simulink model "ford_expedition_cosimulation"  (R2021b)
settings: Solver=ode45  StartTime=0.0  StopTime=45  FixedStep=0.01  RelTol=1e-3  EnableMultiTasking=on
libraries: instrumentlib x2, slpidlib x1
settings Model: PacingRate=11  Creator=tasora  LastModifiedBy=Trevor
settings SolverCC: AlgebraicLoopSolver=TrustRegion
settings DataIOCC: LimitDataPoints=on  SaveFormat=Array  SignalLoggingSaveFormat=ModelDataLogs  ReturnWorkspaceOutputs=off
settings OptimizationCC: ExpressionDepthLimit=2147483647  LifeSpan=inf
settings DebuggingCC: UnderspecifiedInitializationDetection=Classic  MergeDetectMultiDrivingBlocksExec=none  SolverPrmCheckMsg=warning  FcnCallInpInsideContextMsg=warning  StateNameClashWarn=warning  SFUnexpectedBacktrackingDiag=warning  SFNoUnconditionalDefaultTransitionDiag=warning  SFExecutionAtInitializationDiag=none  SFMachineParentedDataDiag=warning  ArithmeticOperatorsInVariantConditions=warning
settings HardwareCC: ProdBitPerPointer=32  ProdBitPerSizeT=32  ProdBitPerPtrDiffT=32  ProdLargestAtomicFloat=None  ProdIntDivRoundTo=Undefined  ProdEndianess=Unspecified  ProdWordSize=32  ProdHWDeviceType=32-bit Generic
settings ModelReferenceCC: PropagateSignalLabelsOutOfModel=off
settings SFSimCC: SimUseLocalCustomCode=off  CustomCodeUndefinedFunction=UseInterfaceOnly
settings RTWCC: RTWUseLocalCustomCode=off
settings CodeAppCC: StateflowObjectComments=on
settings GRTTargetCC: TargetLangStandard=C89/C90 (ANSI)  CombineOutputUpdateFcns=off  GRTInterface=on
settings ConfigComp: CovMetricSettings=dw  CovSaveCumulativeToWorkspaceVar=on  CovSaveSingleToWorkspaceVar=on  CovExternalEMLEnable=off

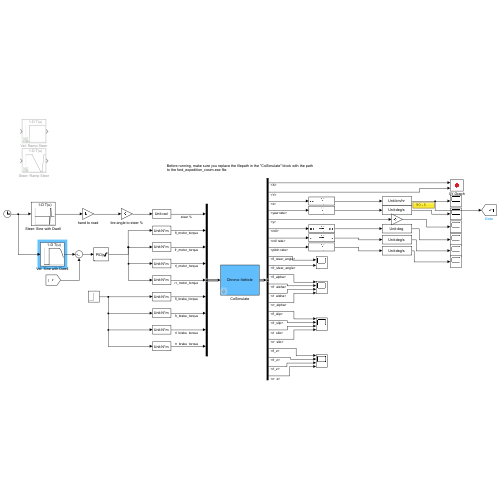
[thumbnail: Simulink's stored preview of the top-level diagram]
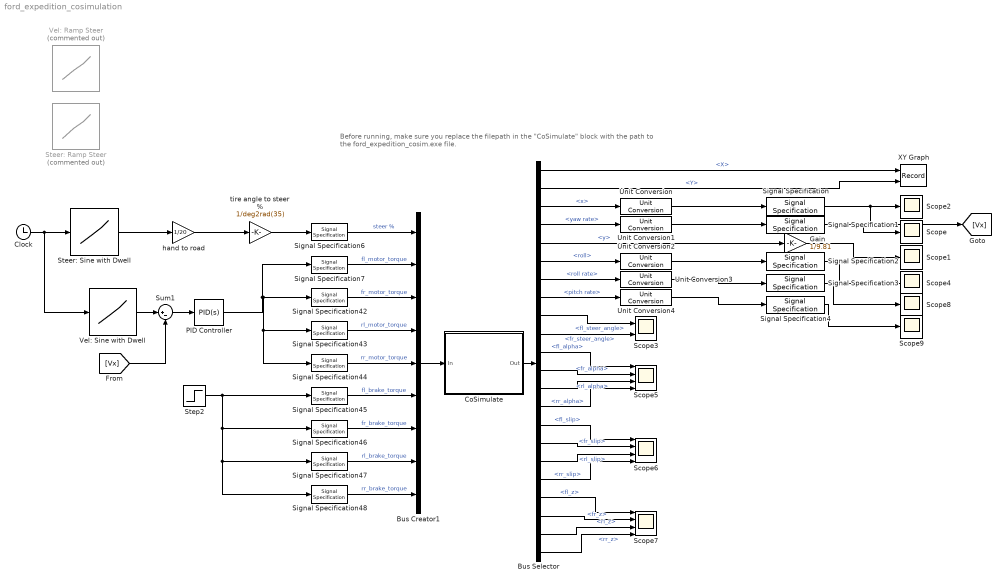
== system ford_expedition_cosimulation ==
  note: Before running, make sure you replace the filepath in the "CoSimulate" block with the path to the ford_expedition_cosim.exe file.
  Bus Creator1 : BusCreator  Inputs=9
  Bus Selector : BusSelector  OutputSignals=global frame.position.X,global frame.position.Y,chassis frame.velocity.x,chassis frame.rotational velocity.yaw rate,chassis frame.acceleration.y,chassis frame.rotation.roll,chassis frame.rotational velocity.roll rate,chassis frame.rotational velocity.pitch rate,inputs.steer angle.fl_steer_angle,inputs.steer angle.fr_steer_angle,wheels.lateral slip.fl_alpha,wheels.lateral slip.fr_alpha,wheels.lateral slip.rl_alpha,wheels.lateral slip.rr_alpha,wheels.longitudinal slip.fl_slip,wheels.longitudinal slip.fr_slip,wheels.longitudinal slip.rl_slip,wheels.longitudinal slip.rr_slip,wheels.vertical force.fl_z,wheels.vertical force.fr_z,wheels.vertical force.rl_z,wheels.vertical force.rr_z
  Clock : Clock
  CoSimulate : Subsystem  Description=|  mask{com_step=1e-2, tcp_data_size=55, host_name=localhost, tcp_port=50009, tcp_timeout=5, exec_path=C:\Users\15309\Project_Chrono\chrono_simulink_cosim\build\Release\cosim_ford_expedition_2003.exe}
      | This block can be used to exchange data with Chrono::Engine.                                                                                      
      | A Chrono::Engine program with a running ChCosimulation inferface must be started, it will work as a server; then the Simulink program must be run.
      | Note! check that the dimensions of the exchanged vectors do match!
      mask prompts: com_step "Communication step size"; tcp_data_size "N. of scalars received from C::E (as block output)"; host_name "TCP host name (ex. 'localhost', or 'www.myhost.com')"; tcp_port "TCP port (ex. 50007)"; tcp_timeout "TCP timeout (seconds)"; exec_path "Executable Path:"
      mask init:
      | block_receive = [gcb, '/TCP Receive'];
      | set_param(block_receive, 'SampleTime', num2str(com_step));
      | set_param(block_receive, 'Host', host_name);
      | set_param(block_receive, 'Port', num2str(tcp_port));
      | set_param(block_receive, 'DataSize', num2str(tcp_data_size+1));
      | set_param(block_receive, 'Timeout', num2str(tcp_timeout));
      | block_send = [gcb, '/TCP Send'];
      | set_param(block_send, 'Host', host_name);
      | set_param(block_send, 'Port', num2str(tcp_port));
      | 
      | % Set the executable extension depending on the OS.
      | if ismac
      |     error("This model cannot run on Mac devices");
      | elseif isunix
      |     extension = "";
      | elseif ispc
      |     extension = ".exe";
      | else
      |     error("Platform not supported")
      | end
      | 
      | % Run Chrono::Vehicle executable.
      | if ~isstring(exec_path)
      |     exec_path = string(exec_path);
      | end
      | if ~isfile(exec_path)
      |     error("The file: '%s', cannot be found.",exec_path);
      | end
      | system(['"', char(exec_path),'" ',num2str(tcp_port),' &']);
      | 
      | % Wait for the executable to establish the TCP server.
      | pause(1.0);
      mask DialogControl Control2 Prompt: Enter below the filepath to the Chrono::Vehicle executable you want to run. In Windows, you can do this:
      mask DialogControl Control4 Prompt: 1. Locate the ".exe" file in File Explorer.
      mask DialogControl Control5 Prompt: 2. Right-click on the executable (ends with ".exe") and select "Copy as Path".
      mask DialogControl Control3 Prompt: 3. Paste the path below.
      mask DialogControl file_path Prompt: Choose cosim executable
      mask DialogControl file_path Callback:
      | [file,path] = uigetfile("*.exe");
      | file_path = string([path,file]);
      | set_param(gcb,'exec_path',file_path);
      mask Display: disp('Chrono::Vehicle')
  Gain : Gain  Gain=1/9.81
  PID Controller : slpidlib/PID Controller  Controller=PID  Form=Parallel  TimeDomain=Continuous-time  UseExternalTs=off  SampleTime=-1  IntegratorMethod=Forward Euler  FilterMethod=Forward Euler  ControllerParametersSource=internal  P=20  I=3  D=1  UseFilter=on  N=100  TunerSelectOption=Transfer Function Based (PID Tuner App)  InitialConditionSource=internal  InitialConditionForIntegrator=0  InitialConditionForFilter=0  DifferentiatorICPrevScaledInput=0  ExternalReset=none  TrackingMode=off  Kt=1  LimitOutput=on  SatLimitsSource=internal  UpperSaturationLimit=800  LowerSaturationLimit=0  LinearizeAsGain=on  AntiWindupMode=back-calculation  Kb=1  POutMin=[]  POutMax=[]  IOutMin=[]  IOutMax=[]  DOutMin=[]  DOutMax=[]  NOutMin=[]  NOutMax=[]  SumOutMin=[]  SumOutMax=[]  SaturationOutMin=[]  SaturationOutMax=[]  PParamMin=[]  PParamMax=[]  IParamMin=[]  IParamMax=[]  DParamMin=[]  DParamMax=[]  NParamMin=[]  NParamMax=[]  KbParamMin=[]  KbParamMax=[]  KtParamMin=[]  KtParamMax=[]  KbOutMin=[]  KbOutMax=[]  KtOutMin=[]  KtOutMax=[]  IntegratorOutMin=[]  IntegratorOutMax=[]  FilterOutMin=[]  FilterOutMax=[]  SumI1OutMin=[]  SumI1OutMax=[]  SumI2OutMin=[]  SumI2OutMax=[]  SumI3OutMin=[]  SumI3OutMax=[]  SumI4OutMin=[]  SumI4OutMax=[]  SumDOutMin=[]  SumDOutMax=[]  DifferentiatorOutMin=[]  DifferentiatorOutMax=[]  FilterDiffOutCoefMin=[]  FilterDiffOutCoefMax=[]  ReciprocalOutMin=[]  ReciprocalOutMax=[]  SumDenOutMin=[]  SumDenOutMax=[]  SumNumOutMin=[]  SumNumOutMax=[]  DivideOutMin=[]  DivideOutMax=[]  UdiffTsProdOutMin=[]  UdiffTsProdOutMax=[]  NTsProdOutMin=[]  NTsProdOutMax=[]  UintegralTsProdOutMin=[]  UintegralTsProdOutMax=[]  UngainTsProdOutMin=[]  UngainTsProdOutMax=[]  IntegratorContinuousStateAttributes=''  IntegratorStateMustResolveToSignalObject=off  IntegratorRTWStateStorageClass=Auto  FilterContinuousStateAttributes=''  FilterStateMustResolveToSignalObject=off  FilterRTWStateStorageClass=Auto  ParallelPVariant=InternalParameters  IdealPVariant=Disabled  IVariant=InternalParameters  DVariant=InternalParameters  IntegratorVariant=Continuous  SatVariant=Enabled  AWVariant=BackCalculation  PCopyVariant=Disabled  TRVariant=Disabled  FdbkBlocksVariant=Forward  IdealPFdbkVariant=Disabled  SatFdbkVariant=Disabled  DerivativeFilterVariant=ContFilter  NVariant=InternalParameters  NCopyVariant=Disabled  FilterICVariant=InternalICsFilter  IntegratorICVariant=InternalICs  ExternalResetVariant=Disabled  TRSumVariant=Passthrough  SumFdbkVariant=Disabled  SumVariant=Sum_PID  TsampFilterVariant=InternalTs  TsampNgainVariant=Passthrough  TsampIntegralVariant=Passthrough  ExternalSaturationOutDataTypeStr=Inherit: Same as second input
  Scope{,1..2,4,8..9} (6 alike) : Scope
  Scope3 : Scope  NumInputPorts=2
  Scope5 : Scope  NumInputPorts=4
  Scope6 : Scope  NumInputPorts=4
  Scope7 : Scope  NumInputPorts=4
  Signal Specification : SignalSpecification  Unit=km/hr
  Signal Specification1 : SignalSpecification  Unit=deg/s
  Signal Specification2 : SignalSpecification  Unit=deg
  Signal Specification3 : SignalSpecification  Unit=deg/s
  Signal Specification4 : SignalSpecification  Unit=deg/s
  Signal Specification{7,42..48} (8 alike) : SignalSpecification  Unit=N*m
  Signal Specification6 : SignalSpecification  Unit=rad
  Steer: Ramp Steer : Lookup_n-D  Commented=on  NumberOfTableDimensions=1  BreakpointsForDimension1=[0, 15, 35, 38, 43, 45]  Table=deg2rad([0, 0, -270, -270, 0, 0])  InternalRulePriority=Speed  RndMeth=Simplest  InputSameDT=on
  Steer: Sine with Dwell : Lookup_n-D  NumberOfTableDimensions=1  BreakpointsForDimension1=[0, 15, 15.08, 15.42, 16.1, 16.67, 17, 20]  Table=deg2rad([0, 0, 1., -160, 160, 160, 0, 0])  InternalRulePriority=Speed  RndMeth=Simplest  InputSameDT=on
  Step2 : Step  Time=45  After=2000  SampleTime=0
  Sum1 : Sum  Inputs=|+-
  Unit Conversion{,1..4} (5 alike) : UnitConversion
  Vel: Ramp Steer : Lookup_n-D  Commented=on  NumberOfTableDimensions=1  BreakpointsForDimension1=[0, 5, 5.01, 15, 25]  Table=[0, 0, 80, 80, 80]  InternalRulePriority=Speed  RndMeth=Simplest  InputSameDT=on
  Vel: Sine with Dwell : Lookup_n-D  NumberOfTableDimensions=1  BreakpointsForDimension1=[0, 5, 5.01, 15, 16, 17, 18, 19, 20]  Table=[0, 0, 80, 80, 79, 72, 63, 50, 35]  InternalRulePriority=Speed  RndMeth=Simplest  InputSameDT=on
  XY Graph : Record  FileSettingsInternal="{\"entries\":[{\"content\":{\"excelSettings\":{\"content\":{},\"type\":\"Streamout.ExcelSettings\"}},\"type\":\"Streamout.FileSettingStorage\",\"uuid\":\"315fc982-1119-45b9-a1ac-29dc23a63e34\"}],\"packageUris\":[\"http://schema.mathworks.com/mf0/streamout_blocks/R2020a\"],\"version\":\"1.0\"}"  Layout=[1 1]  SignalsInternal="{\"entries\":[{\"content\":{\"signals\":[{\"content\":{\"blockPath\":[\"ford_expedition_cosimulation/XY Graph\"],\"channel\":[],\"dimensions\":[1,1],\"domain\":\"ford_expedition_cosimulation/XY Graph\",\"lineColor\":\"#a2142f\",\"plots\":[1],\"port\":1,\"sid\":[\"\"],\"signalID\":96109,\"signalName\":\"<X>\"},\"type\":\"RecordBlkView.Signal\",\"uuid\":\"ad6cb5d7-9066-4b59-9866-374e99120b86\"},{\"content\":{\"blockPath\":[\"ford_expedition_cosimulation/XY Graph\"],\"channel\":[],\"dimensions\":[1,1],\"domain\":\"ford_expedition_cosimulation/XY Graph\",\"lineColor\":\"#139fff\",\"plots\":[1],\"port\":2,\"sid\":[\"\"],\"signalID\":96113,\"signalName\":\"<Y>\"},\"type\":\"RecordBlkView.Signal\",\"uuid\":\"f3f4d94f-e36f-440e-ae2e-7d3cf2cef22d\"}]},\"type\":\"RecordBlkView.InputSignals\",\"uuid\":\"a834540c-b967-49e9-96e8-32a6f391266d\"}],\"packageUris\":[\"http://schema.mathworks.com/mf0/streamout_blocks/R2020a\"],\"version\":\"1.0\"}"  VisualizationBindings="{\"xyplotplugin\":{\"info\":[{\"series\":[{\"bindingParametersList\":[{\"parameter\":\"X-Axis\",\"signalID\":96109,\"signalName\":\"<X>\"},{\"parameter\":\"Y-Axis\",\"signalID\":96113,\"signalName\":\"<Y>\"}],\"seriesID\":13008}],\"subplotID\":1}]}}"  CompatibilityTag=XY
  hand to road : Gain  Gain=1/20
  tire angle to steer % : Gain  Gain=1/deg2rad(35)
  wires:
  Bus Creator1/1 -> CoSimulate/1(In)
  CoSimulate/1(Out) -> Bus Selector/1
  Bus Selector/1 -> XY Graph/1  "<X>"
  Bus Selector/2 -> XY Graph/2  "<Y>"
  Bus Selector/4 -> Unit Conversion1/1  "<yaw rate>"
  Bus Selector/3 -> Unit Conversion/1  "<x>"
  Unit Conversion/1 -> Signal Specification/1
  Signal Specification/1 -> [Vx], Scope2/1
  Unit Conversion1/1 -> Signal Specification1/1
  Signal Specification1/1 -> Scope/1
  Signal Specification48/1 -> Bus Creator1/9  "rr_brake_torque"
  Step2/1 -> Signal Specification45/1, Signal Specification46/1, Signal Specification48/1, Signal Specification47/1
  Signal Specification42/1 -> Bus Creator1/3  "fr_motor_torque"
  Signal Specification6/1 -> Bus Creator1/1  "steer %"
  Signal Specification45/1 -> Bus Creator1/6  "fl_brake_torque"
  Signal Specification7/1 -> Bus Creator1/2  "fl_motor_torque"
  Signal Specification47/1 -> Bus Creator1/8  "rl_brake_torque"
  Signal Specification43/1 -> Bus Creator1/4  "rl_motor_torque"
  Signal Specification44/1 -> Bus Creator1/5  "rr_motor_torque"
  Signal Specification46/1 -> Bus Creator1/7  "fr_brake_torque"
  Bus Selector/5 -> Gain/1  "<y>"
  Bus Selector/9 -> Scope3/1  "<fl_steer_angle>"
  Bus Selector/10 -> Scope3/2  "<fr_steer_angle>"
  tire angle to steer %/1 -> Signal Specification6/1
  hand to road/1 -> tire angle to steer %/1
  PID Controller/1 -> Signal Specification7/1, Signal Specification44/1, Signal Specification43/1, Signal Specification42/1
  Bus Selector/6 -> Unit Conversion2/1  "<roll>"
  Unit Conversion2/1 -> Signal Specification2/1
  Signal Specification2/1 -> Scope4/1
  Bus Selector/11 -> Scope5/1  "<fl_alpha>"
  Bus Selector/12 -> Scope5/2  "<fr_alpha>"
  Bus Selector/13 -> Scope5/3  "<rl_alpha>"
  Bus Selector/14 -> Scope5/4  "<rr_alpha>"
  Gain/1 -> Scope1/1
  Bus Selector/15 -> Scope6/1  "<fl_slip>"
  Bus Selector/16 -> Scope6/2  "<fr_slip>"
  Bus Selector/17 -> Scope6/3  "<rl_slip>"
  Bus Selector/18 -> Scope6/4  "<rr_slip>"
  Bus Selector/19 -> Scope7/1  "<fl_z>"
  Bus Selector/20 -> Scope7/2  "<fr_z>"
  Bus Selector/21 -> Scope7/3  "<rl_z>"
  Bus Selector/22 -> Scope7/4  "<rr_z>"
  Clock/1 -> Vel: Sine with Dwell/1, Steer: Sine with Dwell/1
  Steer: Sine with Dwell/1 -> hand to road/1
  [Vx] -> Sum1/2
  Sum1/1 -> PID Controller/1
  Vel: Sine with Dwell/1 -> Sum1/1
  Signal Specification3/1 -> Scope8/1
  Bus Selector/7 -> Unit Conversion3/1  "<roll rate>"
  Unit Conversion3/1 -> Signal Specification3/1
  Signal Specification4/1 -> Scope9/1
  Bus Selector/8 -> Unit Conversion4/1  "<pitch rate>"
  Unit Conversion4/1 -> Signal Specification4/1

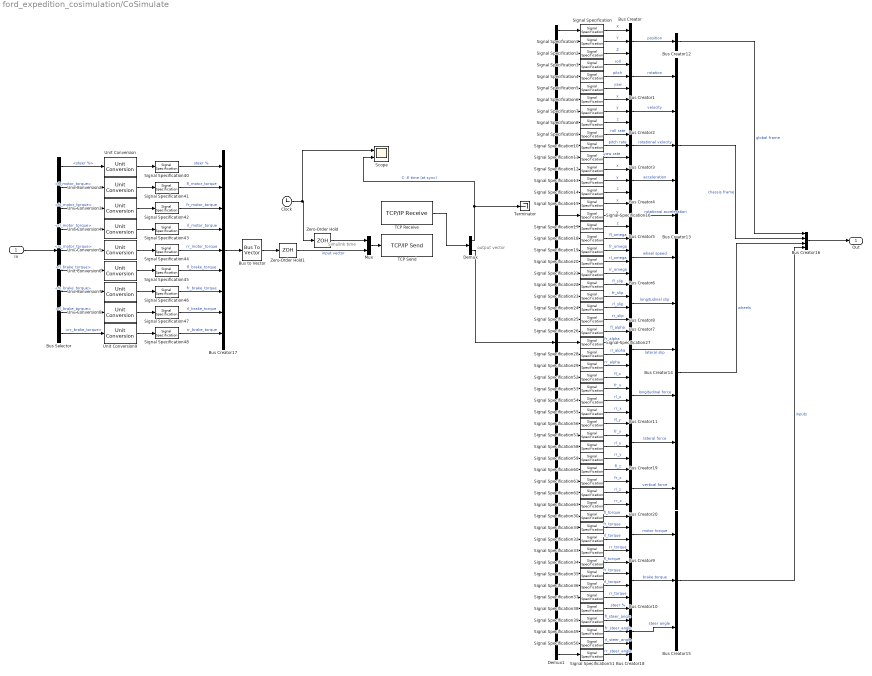
== system ford_expedition_cosimulation/CoSimulate ==
  note: output vector
  note: Simulink time
  In : Inport
  Bus Creator{,1..5,15} (7 alike) : BusCreator  Inputs=3
  Bus Creator{6..11,16,19..20} (9 alike) : BusCreator  Inputs=4
  Bus Creator12 : BusCreator  Inputs=1
  Bus Creator13 : BusCreator  Inputs=5
  Bus Creator14 : BusCreator  Inputs=6
  Bus Creator17 : BusCreator  Inputs=9
  Bus Creator18 : BusCreator  Inputs=5
  Bus Selector : BusSelector  OutputSignals=steer %,fl_motor_torque,fr_motor_torque,rl_motor_torque,rr_motor_torque,fl_brake_torque,fr_brake_torque,rl_brake_torque,rr_brake_torque
  Bus to Vector : BusToVector
  Clock : Clock
  Demux : Demux  Outputs=[1 -1]
  Demux1 : Demux  Outputs=55
  Mux : Mux  Inputs=2
  Scope : Scope  NumInputPorts=2
  Signal Specification : SignalSpecification  Unit=m
  Signal Specification1 : SignalSpecification  Unit=m
  Signal Specification{9..11,18..21} (7 alike) : SignalSpecification  Unit=rad/s
  Signal Specification12 : SignalSpecification  Unit=m/s^2
  Signal Specification13 : SignalSpecification  Unit=m/s^2
  Signal Specification14 : SignalSpecification  Unit=m/s^2
  Signal Specification15 : SignalSpecification  Unit=rad/s^2
  Signal Specification16 : SignalSpecification  Unit=rad/s^2
  Signal Specification17 : SignalSpecification  Unit=rad/s^2
  Signal Specification2 : SignalSpecification  Unit=m
  Signal Specification{22..25} (4 alike) : SignalSpecification  Unit=1
  Signal Specification{3..5,26..29,38..40,49..51} (13 alike) : SignalSpecification  Unit=rad
  Signal Specification{30..37,41..48} (16 alike) : SignalSpecification  Unit=N*m
  Signal Specification{52..63} (12 alike) : SignalSpecification  Unit=N
  Signal Specification6 : SignalSpecification  Unit=m/s
  Signal Specification7 : SignalSpecification  Unit=m/s
  Signal Specification8 : SignalSpecification  Unit=m/s
  TCP Receive : instrumentlib/TCP//IP Receive  Priority=3  Host=localhost  Port=50009  DataSize=56  DataType=double  ASCIIFormatting=%f  Terminator=LF  CustomTerminator=10  ByteOrder=little-endian  EnableBlockingMode=on  Timeout=5  SampleTime=0.01  SimulateUsing=Interpreted execution
  TCP Send : instrumentlib/TCP//IP Send  Priority=2  Host=localhost  Port=50009  ByteOrder=little-endian  EnableBlockingMode=off  Timeout=10  TransferDelay=on  SimulateUsing=Interpreted execution
  Terminator : Terminator
  Unit Conversion{,2..9} (9 alike) : UnitConversion
  Zero-Order Hold : ZeroOrderHold  SampleTime=com_step
  Zero-Order Hold1 : ZeroOrderHold  SampleTime=com_step
  Out : Outport
  wires:
  Zero-Order Hold/1 -> Mux/1
  Zero-Order Hold1/1 -> Mux/2  "input vector"
  Mux/1 -> TCP Send/1
  Clock/1 -> Scope/1, Zero-Order Hold/1
  In/1 -> Bus Selector/1
  TCP Receive/1 -> Demux/1
  Demux/1 -> Scope/2, Terminator/1  "C::E time (at sync)"
  Demux/2 -> Demux1/1
  Demux1/4 -> Signal Specification3/1
  Demux1/1 -> Signal Specification/1
  Demux1/3 -> Signal Specification2/1
  Demux1/10 -> Signal Specification9/1
  Demux1/2 -> Signal Specification1/1
  Demux1/7 -> Signal Specification6/1
  Demux1/11 -> Signal Specification10/1
  Demux1/9 -> Signal Specification8/1
  Demux1/5 -> Signal Specification4/1
  Demux1/6 -> Signal Specification5/1
  Demux1/12 -> Signal Specification11/1
  Demux1/8 -> Signal Specification7/1
  Signal Specification/1 -> Bus Creator/1  "X"
  Signal Specification1/1 -> Bus Creator/2  "Y"
  Signal Specification2/1 -> Bus Creator/3  "Z"
  Signal Specification3/1 -> Bus Creator1/1  "roll"
  Signal Specification4/1 -> Bus Creator1/2  "pitch"
  Signal Specification5/1 -> Bus Creator1/3  "yaw"
  Signal Specification6/1 -> Bus Creator2/1  "x"
  Signal Specification7/1 -> Bus Creator2/2  "y"
  Signal Specification8/1 -> Bus Creator2/3  "z"
  Signal Specification9/1 -> Bus Creator3/1  "roll rate"
  Signal Specification10/1 -> Bus Creator3/2  "pitch rate"
  Signal Specification11/1 -> Bus Creator3/3  "yaw rate"
  Demux1/13 -> Signal Specification12/1
  Demux1/15 -> Signal Specification14/1
  Demux1/14 -> Signal Specification13/1
  Signal Specification12/1 -> Bus Creator4/1  "x"
  Signal Specification13/1 -> Bus Creator4/2  "y"
  Signal Specification14/1 -> Bus Creator4/3  "z"
  Demux1/16 -> Signal Specification15/1
  Demux1/17 -> Signal Specification16/1
  Demux1/18 -> Signal Specification17/1
  Signal Specification15/1 -> Bus Creator5/1  "x"
  Signal Specification16/1 -> Bus Creator5/2  "y"
  Signal Specification17/1 -> Bus Creator5/3  "z"
  Demux1/19 -> Signal Specification18/1
  Demux1/20 -> Signal Specification19/1
  Demux1/21 -> Signal Specification20/1
  Demux1/22 -> Signal Specification21/1
  Signal Specification21/1 -> Bus Creator6/4  "rr_omega"
  Signal Specification20/1 -> Bus Creator6/3  "rl_omega"
  Signal Specification19/1 -> Bus Creator6/2  "fr_omega"
  Signal Specification18/1 -> Bus Creator6/1  "fl_omega"
  Demux1/23 -> Signal Specification22/1
  Demux1/24 -> Signal Specification23/1
  Demux1/26 -> Signal Specification25/1
  Demux1/25 -> Signal Specification24/1
  Signal Specification22/1 -> Bus Creator7/1  "fl_slip"
  Signal Specification23/1 -> Bus Creator7/2  "fr_slip"
  Signal Specification24/1 -> Bus Creator7/3  "rl_slip"
  Signal Specification25/1 -> Bus Creator7/4  "rr_slip"
  Demux1/27 -> Signal Specification26/1
  Demux1/28 -> Signal Specification27/1
  Demux1/29 -> Signal Specification28/1
  Demux1/30 -> Signal Specification29/1
  Signal Specification26/1 -> Bus Creator8/1  "fl_alpha"
  Signal Specification27/1 -> Bus Creator8/2  "fr_alpha"
  Signal Specification28/1 -> Bus Creator8/3  "rl_alpha"
  Signal Specification29/1 -> Bus Creator8/4  "rr_alpha"
  Bus Creator/1 -> Bus Creator12/1  "position"
  Bus Creator1/1 -> Bus Creator13/1  "rotation"
  Bus Creator2/1 -> Bus Creator13/2  "velocity"
  Bus Creator3/1 -> Bus Creator13/3  "rotational velocity"
  Bus Creator4/1 -> Bus Creator13/4  "acceleration"
  Bus Creator5/1 -> Bus Creator13/5  "rotational acceleration"
  Bus Creator6/1 -> Bus Creator14/1  "wheel speed"
  Bus Creator7/1 -> Bus Creator14/2  "longitudinal slip"
  Bus Creator8/1 -> Bus Creator14/3  "lateral slip"
  Bus Creator14/1 -> Bus Creator16/3  "wheels"
  Bus Creator12/1 -> Bus Creator16/1  "global frame"
  Bus Creator13/1 -> Bus Creator16/2  "chassis frame"
  Bus Creator16/1 -> Out/1
  Bus to Vector/1 -> Zero-Order Hold1/1
  Bus Creator17/1 -> Bus to Vector/1
  Signal Specification40/1 -> Bus Creator17/1  "steer %"
  Unit Conversion/1 -> Signal Specification40/1
  Unit Conversion2/1 -> Signal Specification41/1
  Unit Conversion4/1 -> Signal Specification43/1
  Unit Conversion5/1 -> Signal Specification44/1
  Unit Conversion3/1 -> Signal Specification42/1
  Signal Specification41/1 -> Bus Creator17/2  "fl_motor_torque"
  Signal Specification42/1 -> Bus Creator17/3  "fr_motor_torque"
  Signal Specification43/1 -> Bus Creator17/4  "rl_motor_torque"
  Signal Specification44/1 -> Bus Creator17/5  "rr_motor_torque"
  Signal Specification48/1 -> Bus Creator17/9  "rr_brake_torque"
  Signal Specification47/1 -> Bus Creator17/8  "rl_brake_torque"
  Signal Specification46/1 -> Bus Creator17/7  "fr_brake_torque"
  Signal Specification45/1 -> Bus Creator17/6  "fl_brake_torque"
  Unit Conversion7/1 -> Signal Specification46/1
  Unit Conversion9/1 -> Signal Specification48/1
  Unit Conversion8/1 -> Signal Specification47/1
  Unit Conversion6/1 -> Signal Specification45/1
  Bus Selector/1 -> Unit Conversion/1  "<steer %>"
  Bus Selector/2 -> Unit Conversion2/1  "<fl_motor_torque>"
  Bus Selector/3 -> Unit Conversion3/1  "<fr_motor_torque>"
  Bus Selector/4 -> Unit Conversion4/1  "<rl_motor_torque>"
  Bus Selector/5 -> Unit Conversion5/1  "<rr_motor_torque>"
  Bus Selector/6 -> Unit Conversion6/1  "<fl_brake_torque>"
  Bus Selector/7 -> Unit Conversion7/1  "<fr_brake_torque>"
  Bus Selector/8 -> Unit Conversion8/1  "<rl_brake_torque>"
  Bus Selector/9 -> Unit Conversion9/1  "<rr_brake_torque>"
  Bus Creator18/1 -> Bus Creator15/3  "steer angle"
  Signal Specification50/1 -> Bus Creator18/4  "rl_steer_angle"
  Demux1/55 -> Signal Specification51/1
  Demux1/52 -> Signal Specification39/1
  Bus Creator10/1 -> Bus Creator15/2  "brake torque"
  Demux1/46 -> Signal Specification33/1
  Signal Specification39/1 -> Bus Creator18/2  "fl_steer_angle"
  Signal Specification49/1 -> Bus Creator18/3  "fr_steer_angle"
  Demux1/44 -> Signal Specification31/1
  Signal Specification51/1 -> Bus Creator18/5  "rr_steer_angle"
  Signal Specification35/1 -> Bus Creator10/2  "fr_torque"
  Signal Specification38/1 -> Bus Creator18/1  "steer %"
  Bus Creator9/1 -> Bus Creator15/1  "motor torque"
  Demux1/53 -> Signal Specification49/1
  Bus Creator15/1 -> Bus Creator16/4  "inputs"
  Signal Specification37/1 -> Bus Creator10/4  "rr_torque"
  Demux1/54 -> Signal Specification50/1
  Signal Specification36/1 -> Bus Creator10/3  "rl_torque"
  Demux1/43 -> Signal Specification30/1
  Signal Specification34/1 -> Bus Creator10/1  "fl_torque"
  Demux1/51 -> Signal Specification38/1
  Signal Specification31/1 -> Bus Creator9/2  "fr_torque"
  Signal Specification30/1 -> Bus Creator9/1  "fl_torque"
  Demux1/48 -> Signal Specification35/1
  Signal Specification32/1 -> Bus Creator9/3  "rl_torque"
  Demux1/45 -> Signal Specification32/1
  Demux1/50 -> Signal Specification37/1
  Demux1/49 -> Signal Specification36/1
  Demux1/47 -> Signal Specification34/1
  Signal Specification33/1 -> Bus Creator9/4  "rr_torque"
  Demux1/31 -> Signal Specification52/1
  Demux1/32 -> Signal Specification53/1
  Demux1/33 -> Signal Specification54/1
  Demux1/34 -> Signal Specification55/1
  Signal Specification52/1 -> Bus Creator11/1  "fl_x"
  Signal Specification53/1 -> Bus Creator11/2  "fr_x"
  Signal Specification54/1 -> Bus Creator11/3  "rl_x"
  Signal Specification55/1 -> Bus Creator11/4  "rr_x"
  Demux1/35 -> Signal Specification56/1
  Demux1/38 -> Signal Specification59/1
  Demux1/36 -> Signal Specification57/1
  Demux1/37 -> Signal Specification58/1
  Signal Specification58/1 -> Bus Creator19/3  "rl_y"
  Signal Specification59/1 -> Bus Creator19/4  "rr_y"
  Signal Specification57/1 -> Bus Creator19/2  "fr_y"
  Signal Specification56/1 -> Bus Creator19/1  "fl_y"
  Demux1/39 -> Signal Specification60/1
  Demux1/42 -> Signal Specification63/1
  Demux1/40 -> Signal Specification61/1
  Demux1/41 -> Signal Specification62/1
  Signal Specification62/1 -> Bus Creator20/3  "rl_z"
  Signal Specification63/1 -> Bus Creator20/4  "rr_z"
  Signal Specification61/1 -> Bus Creator20/2  "fr_z"
  Signal Specification60/1 -> Bus Creator20/1  "fl_z"
  Bus Creator11/1 -> Bus Creator14/4  "longitudinal force"
  Bus Creator19/1 -> Bus Creator14/5  "lateral force"
  Bus Creator20/1 -> Bus Creator14/6  "vertical force"
